simulink model "Noordergraaf_Rideout"  (R2022b)
settings: Solver=FixedStepAuto  StartTime=0.0  StopTime=stop_time  FixedStep=sample_time  RelTol=1e-3
InitFcn:
  | init_fcn_noordergraaf_rideout
StopFcn:
  | stop_fcn_noordergraaf_rideout
undefined symbols (not defined in the file): C, Cep, Cev, Cla, Cpa, Cpp, Cpv, Cra, Csa, Csp, Csv, Dx, fcs0, fes0, fes1, fesmin, fev0, fev1, fmax, fmin, Gx, initx, ka, KElv, KErv, kes, kev, KRlv, KRrv, ksys, L, Lpa, Lsa, P0lv, P0rv, Pn, R, R_105, R_26, R_29, R_34, R_35, R_60, R_61, R_64, R_65, R_66, R_70, R_82, R_84, R_88, R_90, R_AT, R_SA, Rev, Rla, Rpa, Rpp, Rpv, Rra ... (+18)
libraries: ee_lib x419, fl_lib x77, nesl_utility x52, simulink x2
(part 9 of 9)

== system Noordergraaf_Rideout/RLC_97 ==
  Capacitor : ee_lib/Passive/Capacitor  cap_option=0  c=C F  Cvec=[1e-05, 1e-06] F  Vvec=[0, 10] V  CV_table_symmetry=1  f_vec=[1, 10] kHz  DFext_vec=[.8, 1.2]  enable_C_tol=0  C_tol=5  tol_distribution=1  nSigma=4  r=1e-6 Ohm  g=0 1/Ohm  averaging_period=0 s  enable_operating_limits=0  operating_limit_action=2  max_working_voltage_range=[-25, 25] V  power_rating=1 W  enable_faults=0  fault_action=1  Cscale_faulted=100  R_faulted=1e-3 Ohm  G_faulted=0 1/Ohm  tau_fault=1e-3 s  enable_temporal_fault=0  t_fault=1 s  enable_behavioral_fault=0  max_permissible_voltage_range=[-100, 100] V  t_fail_on_voltage=1 s  i_specify=off  i_priority=None  i=0 A  i_nominal_specify=off  i_nominal_unit=A  i_nominal_value=1  v_specify=off  v_priority=None  v=0 V  v_nominal_specify=off  v_nominal_unit=V  v_nominal_value=1  vc_specify=off  vc_priority=High  vc=0 V  vc_nominal_specify=off  vc_nominal_unit=V  vc_nominal_value=1
  Inductor : ee_lib/Passive/Inductor  l=L H  enable_L_tol=0  L_tol=20  tol_distribution=1  nSigma=4  r=0 Ohm  g=1e-9 1/Ohm  enable_operating_limits=0  operating_limit_action=2  max_working_current=1 A  power_rating=1 W  enable_faults=0  fault_action=1  lambdaPercent=50  k_faulted=0.9999  turnsShort=0  openCct=0  groundShort=0  groundShortG=0 1/Ohm  tau_fault=1e-3 s  enable_temporal_fault=0  t_fault=1 s  enable_behavioral_fault=0  max_permissible_voltage=100 V  n_fail_on_voltage=1  max_permissible_current=1 A  t_fail_on_current=1 s  i_L_specify=off  i_L_priority=High  i_L=0 A  i_L_nominal_specify=off  i_L_nominal_unit=A  i_L_nominal_value=1
  Resistor1 : ee_lib/Passive/Resistor  R=R Ohm  enable_R_tol=0  R_tol=5  tol_distribution=1  nSigma=4  enable_operating_limits=0  operating_limit_action=2  max_working_voltage=100 V  power_rating=1 W  enable_faults=0  fault_action=1  R_faulted=inf Ohm  enable_temporal_fault=0  t_fault=1 s  enable_behavioral_fault=0  max_permissible_current=1 A  t_fail_on_current=1 s  noise_mode=0  sample_time=1e-3 s  repeatability=1  auto_seed=1874010528  user_seed=0  Tdevice=25 degC  power_derating_T1=70 degC  power_derating_T2=155 degC  operating_temperature_range_vec=[-50, 150] degC  alpha=3.93e-3 1/K  Tmeas=25 degC  thermal_mass=100 J/K  temperature_specify=off  temperature_priority=High  temperature=298.15 K  temperature_nominal_specify=off  temperature_nominal_unit=K  temperature_nominal_value=1
  Out_A : PMIOPort  Side=Left
  Out_B : PMIOPort  Port=2  Side=Left
  In_A : PMIOPort  Port=3  Side=Right
  In_B : PMIOPort  Port=4  Side=Right
  connections:
  Capacitor/LConn1 -- Out_A/RConn1 -- Inductor/RConn1
  Resistor1/RConn1 -- Inductor/LConn1
  Out_B/RConn1 -- In_B/RConn1 -- Capacitor/RConn1
  Resistor1/LConn1 -- In_A/RConn1

== system Noordergraaf_Rideout/RLC_98 ==
  Capacitor : ee_lib/Passive/Capacitor  cap_option=0  c=C F  Cvec=[1e-05, 1e-06] F  Vvec=[0, 10] V  CV_table_symmetry=1  f_vec=[1, 10] kHz  DFext_vec=[.8, 1.2]  enable_C_tol=0  C_tol=5  tol_distribution=1  nSigma=4  r=1e-6 Ohm  g=0 1/Ohm  averaging_period=0 s  enable_operating_limits=0  operating_limit_action=2  max_working_voltage_range=[-25, 25] V  power_rating=1 W  enable_faults=0  fault_action=1  Cscale_faulted=100  R_faulted=1e-3 Ohm  G_faulted=0 1/Ohm  tau_fault=1e-3 s  enable_temporal_fault=0  t_fault=1 s  enable_behavioral_fault=0  max_permissible_voltage_range=[-100, 100] V  t_fail_on_voltage=1 s  i_specify=off  i_priority=None  i=0 A  i_nominal_specify=off  i_nominal_unit=A  i_nominal_value=1  v_specify=off  v_priority=None  v=0 V  v_nominal_specify=off  v_nominal_unit=V  v_nominal_value=1  vc_specify=off  vc_priority=High  vc=0 V  vc_nominal_specify=off  vc_nominal_unit=V  vc_nominal_value=1
  Inductor : ee_lib/Passive/Inductor  l=L H  enable_L_tol=0  L_tol=20  tol_distribution=1  nSigma=4  r=0 Ohm  g=1e-9 1/Ohm  enable_operating_limits=0  operating_limit_action=2  max_working_current=1 A  power_rating=1 W  enable_faults=0  fault_action=1  lambdaPercent=50  k_faulted=0.9999  turnsShort=0  openCct=0  groundShort=0  groundShortG=0 1/Ohm  tau_fault=1e-3 s  enable_temporal_fault=0  t_fault=1 s  enable_behavioral_fault=0  max_permissible_voltage=100 V  n_fail_on_voltage=1  max_permissible_current=1 A  t_fail_on_current=1 s  i_L_specify=off  i_L_priority=High  i_L=0 A  i_L_nominal_specify=off  i_L_nominal_unit=A  i_L_nominal_value=1
  Resistor1 : ee_lib/Passive/Resistor  R=R Ohm  enable_R_tol=0  R_tol=5  tol_distribution=1  nSigma=4  enable_operating_limits=0  operating_limit_action=2  max_working_voltage=100 V  power_rating=1 W  enable_faults=0  fault_action=1  R_faulted=inf Ohm  enable_temporal_fault=0  t_fault=1 s  enable_behavioral_fault=0  max_permissible_current=1 A  t_fail_on_current=1 s  noise_mode=0  sample_time=1e-3 s  repeatability=1  auto_seed=746693110  user_seed=0  Tdevice=25 degC  power_derating_T1=70 degC  power_derating_T2=155 degC  operating_temperature_range_vec=[-50, 150] degC  alpha=3.93e-3 1/K  Tmeas=25 degC  thermal_mass=100 J/K  temperature_specify=off  temperature_priority=High  temperature=298.15 K  temperature_nominal_specify=off  temperature_nominal_unit=K  temperature_nominal_value=1
  Out_A : PMIOPort  Side=Left
  Out_B : PMIOPort  Port=2  Side=Left
  In_A : PMIOPort  Port=3  Side=Right
  In_B : PMIOPort  Port=4  Side=Right
  connections:
  Capacitor/LConn1 -- Out_A/RConn1 -- Inductor/RConn1
  Resistor1/RConn1 -- Inductor/LConn1
  Out_B/RConn1 -- In_B/RConn1 -- Capacitor/RConn1
  Resistor1/LConn1 -- In_A/RConn1

== system Noordergraaf_Rideout/RLC_99 ==
  Capacitor : ee_lib/Passive/Capacitor  cap_option=0  c=C F  Cvec=[1e-05, 1e-06] F  Vvec=[0, 10] V  CV_table_symmetry=1  f_vec=[1, 10] kHz  DFext_vec=[.8, 1.2]  enable_C_tol=0  C_tol=5  tol_distribution=1  nSigma=4  r=1e-6 Ohm  g=0 1/Ohm  averaging_period=0 s  enable_operating_limits=0  operating_limit_action=2  max_working_voltage_range=[-25, 25] V  power_rating=1 W  enable_faults=0  fault_action=1  Cscale_faulted=100  R_faulted=1e-3 Ohm  G_faulted=0 1/Ohm  tau_fault=1e-3 s  enable_temporal_fault=0  t_fault=1 s  enable_behavioral_fault=0  max_permissible_voltage_range=[-100, 100] V  t_fail_on_voltage=1 s  i_specify=off  i_priority=None  i=0 A  i_nominal_specify=off  i_nominal_unit=A  i_nominal_value=1  v_specify=off  v_priority=None  v=0 V  v_nominal_specify=off  v_nominal_unit=V  v_nominal_value=1  vc_specify=off  vc_priority=High  vc=0 V  vc_nominal_specify=off  vc_nominal_unit=V  vc_nominal_value=1
  Inductor : ee_lib/Passive/Inductor  l=L H  enable_L_tol=0  L_tol=20  tol_distribution=1  nSigma=4  r=0 Ohm  g=1e-9 1/Ohm  enable_operating_limits=0  operating_limit_action=2  max_working_current=1 A  power_rating=1 W  enable_faults=0  fault_action=1  lambdaPercent=50  k_faulted=0.9999  turnsShort=0  openCct=0  groundShort=0  groundShortG=0 1/Ohm  tau_fault=1e-3 s  enable_temporal_fault=0  t_fault=1 s  enable_behavioral_fault=0  max_permissible_voltage=100 V  n_fail_on_voltage=1  max_permissible_current=1 A  t_fail_on_current=1 s  i_L_specify=off  i_L_priority=High  i_L=0 A  i_L_nominal_specify=off  i_L_nominal_unit=A  i_L_nominal_value=1
  Resistor1 : ee_lib/Passive/Resistor  R=R Ohm  enable_R_tol=0  R_tol=5  tol_distribution=1  nSigma=4  enable_operating_limits=0  operating_limit_action=2  max_working_voltage=100 V  power_rating=1 W  enable_faults=0  fault_action=1  R_faulted=inf Ohm  enable_temporal_fault=0  t_fault=1 s  enable_behavioral_fault=0  max_permissible_current=1 A  t_fail_on_current=1 s  noise_mode=0  sample_time=1e-3 s  repeatability=1  auto_seed=112129176  user_seed=0  Tdevice=25 degC  power_derating_T1=70 degC  power_derating_T2=155 degC  operating_temperature_range_vec=[-50, 150] degC  alpha=3.93e-3 1/K  Tmeas=25 degC  thermal_mass=100 J/K  temperature_specify=off  temperature_priority=High  temperature=298.15 K  temperature_nominal_specify=off  temperature_nominal_unit=K  temperature_nominal_value=1
  Out_A : PMIOPort  Side=Left
  Out_B : PMIOPort  Port=2  Side=Left
  In_A : PMIOPort  Port=3  Side=Right
  In_B : PMIOPort  Port=4  Side=Right
  connections:
  Capacitor/LConn1 -- Out_A/RConn1 -- Inductor/RConn1
  Resistor1/RConn1 -- Inductor/LConn1
  Out_B/RConn1 -- In_B/RConn1 -- Capacitor/RConn1
  Resistor1/LConn1 -- In_A/RConn1

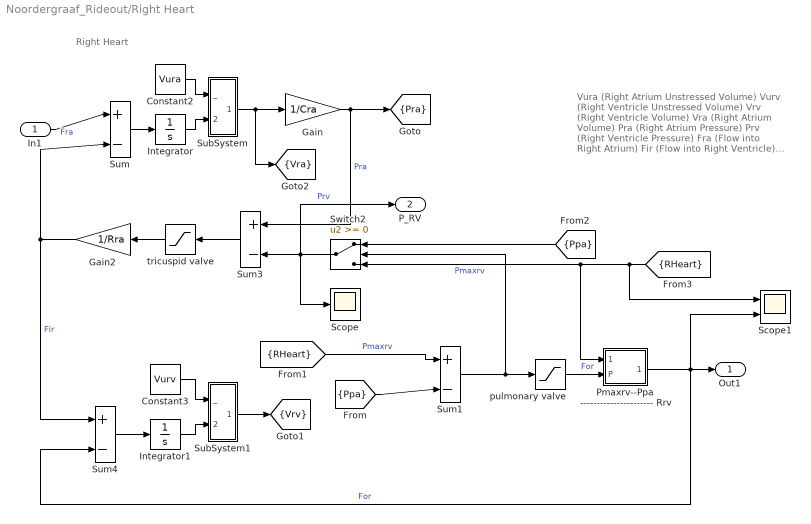
== system Noordergraaf_Rideout/Right Heart ==
  note: Right Heart
  note: Vura (Right Atrium Unstressed Volume)
      | Vurv (Right Ventricle Unstressed Volume)
      | Vrv (Right Ventricle Volume)
      | Vra (Right Atrium Volume)
      | Pra (Right Atrium Pressure)
      | Prv (Right Ventricle Pressure)
      | Fra (Flow into Right Atrium)
      | Fir (Flow into Right Ventricle)
      | For (Flow out of Right Ventricle)
      | LHeart (Left Ventricle Function)
  In1 : Inport
  Constant2 : Constant  Value=Vura
  Constant3 : Constant  Value=Vurv
  Gain : Gain  Gain=1/Cra  SaturateOnIntegerOverflow=on
  Gain2 : Gain  Gain=1/Rra  SaturateOnIntegerOverflow=on
  Integrator : Integrator
  Integrator1 : Integrator
  Pmaxrv--Ppa ---------------------- Rrv : Subsystem
  Scope : Scope
  Scope1 : Scope  NumInputPorts=2
  SubSystem : Subsystem
  SubSystem1 : Subsystem
  Sum : Sum  Inputs=|+-  SaturateOnIntegerOverflow=on
  Sum1 : Sum  Inputs=|+-  SaturateOnIntegerOverflow=on
  Sum3 : Sum  Inputs=+-  SaturateOnIntegerOverflow=on
  Sum4 : Sum  Inputs=+-  SaturateOnIntegerOverflow=on
  Switch2 : Switch
  pulmonary valve : Saturate  UpperLimit=inf  LowerLimit=0
  tricuspid valve : Saturate  UpperLimit=inf  LowerLimit=0
  Out1 : Outport
  P_RV : Outport  Port=2
  tag scope: Pra=scoped, Vra=scoped, Vrv=scoped
  wires:
  In1/1 -> Sum/1  "Fra"
  Sum/1 -> Integrator/1
  [Ppa] -> Sum1/2
  Gain/1 -> [Pra], Sum3/1  "Pra"
  Gain2/1 -> Sum/2, Sum4/1  "Fir"
  Integrator/1 -> SubSystem/2(+)
  Constant2/1 -> SubSystem/1(_)
  SubSystem1/1(Out) -> [Vrv]
  SubSystem/1(Out) -> Gain/1, [Vra]
  Constant3/1 -> SubSystem1/1(_)
  Integrator1/1 -> SubSystem1/2(+)
  [RHeart] -> Sum1/1  "Pmaxrv"
  Sum1/1 -> pulmonary valve/1, Switch2/2
  [Ppa] -> Switch2/1
  tricuspid valve/1 -> Gain2/1
  pulmonary valve/1 -> Pmaxrv--Ppa ---------------------- Rrv/2(P)  "For"
  Pmaxrv--Ppa ---------------------- Rrv/1(Flow) -> Scope1/2, Out1/1, Sum4/2  "For"
  [RHeart] -> Scope1/1, Switch2/3, Pmaxrv--Ppa ---------------------- Rrv/1(Pmax)  "Pmaxrv"
  Sum4/1 -> Integrator1/1
  Sum3/1 -> tricuspid valve/1
  Switch2/1 -> P_RV/1, Sum3/2, Scope/1  "Prv"

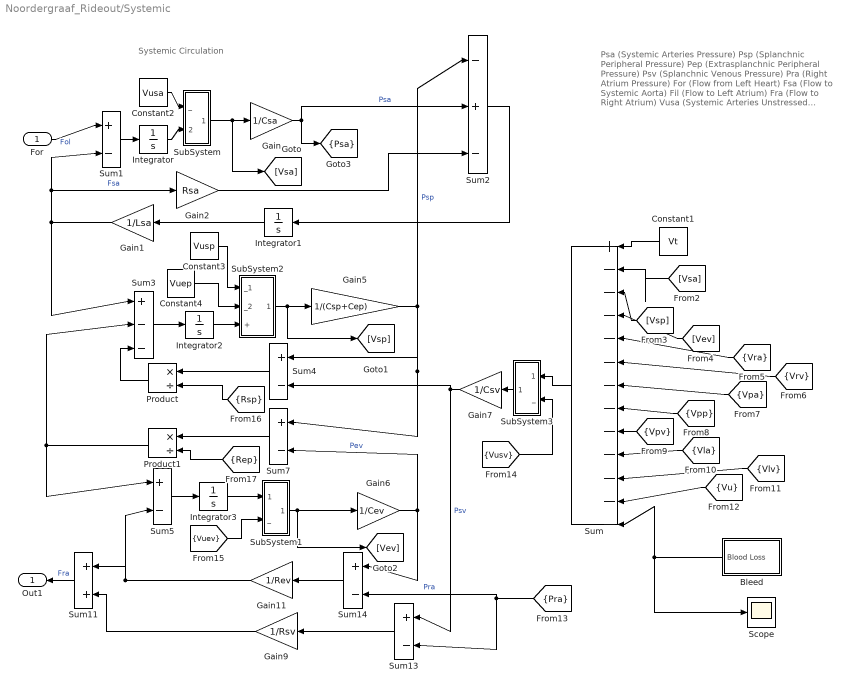
== system Noordergraaf_Rideout/Systemic ==
  note: Psa (Systemic Arteries Pressure)
      | Psp (Splanchnic Peripheral Pressure)
      | Pep (Extrasplanchnic Peripheral Pressure)
      | Psv (Splanchnic Venous Pressure)
      | Pra (Right Atrium Pressure)
      | For (Flow from Left Heart)
      | Fsa (Flow to Systemic Aorta)
      | Fil (Flow to Left Atrium)
      | Fra (Flow to Right Atrium)
      | Vusa (Systemic Arteries Unstressed Volume)
      | Vusp (Extrasplanchnic Venous Unstressed Volume)
      | Vuep (Splanchnic Venous Unstressed Volume)
      | Vuev (Extrasplanchnic Venous Unstressed Volume)
      | Vusv (Splanchnic Venous Unstressed Volume)
  note: Systemic Circulation
  For : Inport
  Bleed : Subsystem  mask{ulimit=0, rate=0, tstart=0}
      mask prompts: ulimit "Bleed Up Limit (ml)"; rate "Bleed Rate (ml/s)"; tstart "Bleed Start Time (s)"
  Constant1 : Constant  Value=Vt
  Constant2 : Constant  Value=Vusa
  Constant3 : Constant  Value=Vusp
  Constant4 : Constant  Value=Vuep
  Gain : Gain  Gain=1/Csa  SaturateOnIntegerOverflow=on
  Gain1 : Gain  Gain=1/Lsa  SaturateOnIntegerOverflow=on
  Gain11 : Gain  Gain=1/Rev  SaturateOnIntegerOverflow=on
  Gain2 : Gain  Gain=Rsa  SaturateOnIntegerOverflow=on
  Gain5 : Gain  Gain=1/(Csp+Cep)  SaturateOnIntegerOverflow=on
  Gain6 : Gain  Gain=1/Cev  SaturateOnIntegerOverflow=on
  Gain7 : Gain  Gain=1/Csv  SaturateOnIntegerOverflow=on
  Gain9 : Gain  Gain=1/Rsv  SaturateOnIntegerOverflow=on
  Integrator{,1..3} (4 alike) : Integrator
  Product : Product  Inputs=*/  SaturateOnIntegerOverflow=on
  Product1 : Product  Inputs=*/  SaturateOnIntegerOverflow=on
  Scope : Scope
  SubSystem : Subsystem
  SubSystem1 : Subsystem
  SubSystem2 : Subsystem
  SubSystem3 : Subsystem
  Sum : Sum  Inputs=|+------------  SaturateOnIntegerOverflow=on
  Sum{1,4..5,7,13..14} (6 alike) : Sum  Inputs=|+-  SaturateOnIntegerOverflow=on
  Sum11 : Sum  Inputs=|++  SaturateOnIntegerOverflow=on
  Sum2 : Sum  Inputs=|-+-  SaturateOnIntegerOverflow=on
  Sum3 : Sum  Inputs=|+--  SaturateOnIntegerOverflow=on
  Out1 : Outport
  tag scope: Psa=scoped
  wires:
  For/1 -> Sum1/1  "Fol"
  Sum1/1 -> Integrator/1
  Integrator1/1 -> Gain1/1
  Sum2/1 -> Integrator1/1
  Gain2/1 -> Sum2/3
  Gain1/1 -> Sum1/2, Gain2/1, Sum3/1  "Fsa"
  Sum3/1 -> Integrator2/1
  Gain5/1 -> Sum2/1, Sum4/1, Sum7/1  "Psp"
  Product/1 -> Sum3/3
  Product1/1 -> Sum3/2, Sum5/1
  Integrator3/1 -> SubSystem1/1(+)
  SubSystem1/1(Out) -> Gain6/1, [Vev]
  Constant1/1 -> Sum/1
  [Vsa] -> Sum/2
  [Vsp] -> Sum/3
  [Vev] -> Sum/4
  [Vra] -> Sum/5
  [Vrv] -> Sum/6
  [Vpa] -> Sum/7
  [Vpp] -> Sum/8
  [Vpv] -> Sum/9
  [Vla] -> Sum/10
  [Vlv] -> Sum/11
  [Vu] -> Sum/12
  Integrator/1 -> SubSystem/2(+)
  SubSystem/1(Out) -> Gain/1, [Vsa]
  Integrator2/1 -> SubSystem2/3(+)
  SubSystem2/1(Out) -> Gain5/1, [Vsp]
  SubSystem3/1(Out) -> Gain7/1
  Sum13/1 -> Gain9/1
  Sum11/1 -> Out1/1  "Fra"
  Gain7/1 -> Sum4/2, Sum13/1  "Psv"
  Gain9/1 -> Sum11/2
  Gain6/1 -> Sum7/2, Sum14/1  "Pev"
  Sum14/1 -> Gain11/1
  [Pra] -> Sum13/2, Sum14/2  "Pra"
  Sum5/1 -> Integrator3/1
  Gain11/1 -> Sum11/1, Sum5/2
  Gain/1 -> [Psa], Sum2/2  "Psa"
  Constant2/1 -> SubSystem/1(_)
  [Vuev] -> SubSystem1/2(_)
  Constant3/1 -> SubSystem2/1(_1)
  Constant4/1 -> SubSystem2/2(_2)
  Sum/1 -> SubSystem3/1(+)
  [Vusv] -> SubSystem3/2(_)
  Sum4/1 -> Product/1
  [Rsp] -> Product/2
  [Rep] -> Product1/2
  Sum7/1 -> Product1/1
  Bleed/1(Blood Loss) -> Sum/13, Scope/1

== system Noordergraaf_Rideout/Voltage Source (SL) ==
  S : Inport
  Controlled Voltage Source : fl_lib/Electrical/Electrical Sources/Controlled Voltage Source
  Simulink-PS Converter : nesl_utility/Simulink-PS Converter  PhysicalDomain=network_engine_domain  SubClassName=ps_input  LeftPortType=input  RightPortType=output  PseudoPeriodic=off  Frequencies=[]  NoiseDistribution=none  NoiseParameters=[]  Unit=V  AffineConversion=off  FilteringAndDerivatives=zero  SimscapeFilterOrder=1  InputFilterTimeConstant=.001  UdotUserProvided=0
  + : PMIOPort  Side=Right
  - : PMIOPort  Port=2  Side=Right
  wires:
  S/1 -> Simulink-PS Converter/1
  connections:
  +/RConn1 -- Controlled Voltage Source/LConn1
  -/RConn1 -- Controlled Voltage Source/RConn2
  Controlled Voltage Source/RConn1 -- Simulink-PS Converter/RConn1

== system Noordergraaf_Rideout/Control/Carotid Sinus ==
  Pin : Inport
  Fcn : Fcn  Expr=(fmin+fmax*exp((u-Pn)/ka))/(1+exp((u-Pn)/ka))
  Transfer Fcn : TransferFcn  Numerator=[touz 1]  Denominator=[toup 1]
  fcs : Outport
  wires:
  Pin/1 -> Transfer Fcn/1
  Transfer Fcn/1 -> Fcn/1
  Fcn/1 -> fcs/1

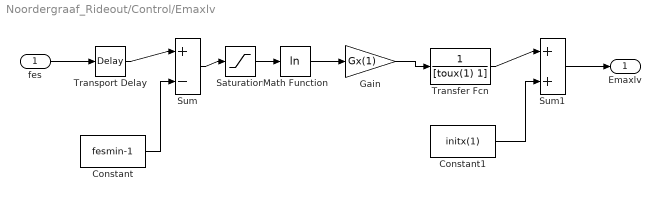
== system Noordergraaf_Rideout/Control/Emaxlv ==
  fes : Inport
  Constant : Constant  Value=fesmin-1
  Constant1 : Constant  Value=initx(1)
  Gain : Gain  Gain=Gx(1)  SaturateOnIntegerOverflow=on
  Math Function : Math  Operator=log
  Saturation : Saturate  UpperLimit=inf  LowerLimit=1
  Sum : Sum  Inputs=|+-  SaturateOnIntegerOverflow=on
  Sum1 : Sum  Inputs=|++  SaturateOnIntegerOverflow=on
  Transfer Fcn : TransferFcn  Denominator=[toux(1) 1]
  Transport Delay : TransportDelay  DelayTime=Dx(1)
  Emaxlv : Outport
  wires:
  fes/1 -> Transport Delay/1
  Transport Delay/1 -> Sum/1
  Constant/1 -> Sum/2
  Sum/1 -> Saturation/1
  Saturation/1 -> Math Function/1
  Math Function/1 -> Gain/1
  Gain/1 -> Transfer Fcn/1
  Transfer Fcn/1 -> Sum1/1
  Sum1/1 -> Emaxlv/1
  Constant1/1 -> Sum1/2

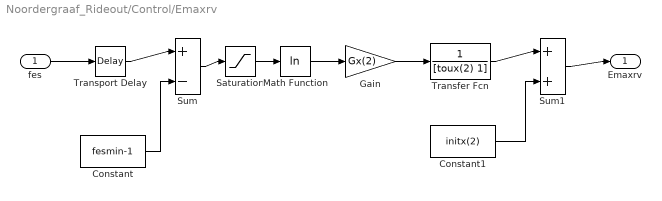
== system Noordergraaf_Rideout/Control/Emaxrv ==
  fes : Inport
  Constant : Constant  Value=fesmin-1
  Constant1 : Constant  Value=initx(2)
  Gain : Gain  Gain=Gx(2)  SaturateOnIntegerOverflow=on
  Math Function : Math  Operator=log
  Saturation : Saturate  UpperLimit=inf  LowerLimit=1
  Sum : Sum  Inputs=|+-  SaturateOnIntegerOverflow=on
  Sum1 : Sum  Inputs=|++  SaturateOnIntegerOverflow=on
  Transfer Fcn : TransferFcn  Denominator=[toux(2) 1]
  Transport Delay : TransportDelay  DelayTime=Dx(2)
  Emaxrv : Outport
  wires:
  Constant1/1 -> Sum1/2
  Sum1/1 -> Emaxrv/1
  Transfer Fcn/1 -> Sum1/1
  Gain/1 -> Transfer Fcn/1
  Math Function/1 -> Gain/1
  Saturation/1 -> Math Function/1
  Sum/1 -> Saturation/1
  Constant/1 -> Sum/2
  Transport Delay/1 -> Sum/1
  fes/1 -> Transport Delay/1

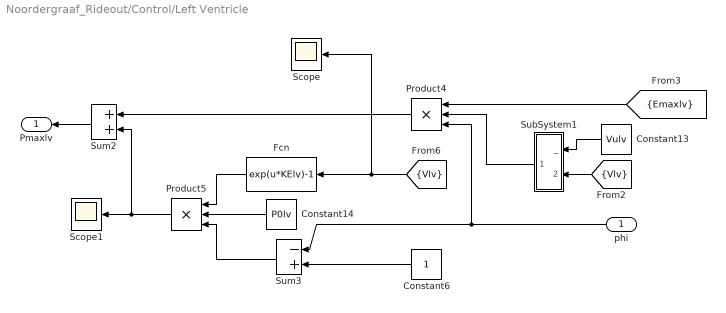
== system Noordergraaf_Rideout/Control/Left Ventricle ==
  phi : Inport
  Constant13 : Constant  Value=Vulv
  Constant14 : Constant  Value=P0lv
  Constant6 : Constant
  Fcn : Fcn  Expr=exp(u*KElv)-1
  Product4 : Product  Inputs=3  SaturateOnIntegerOverflow=on
  Product5 : Product  Inputs=3  SaturateOnIntegerOverflow=on
  Scope : Scope
  Scope1 : Scope
  SubSystem1 : Subsystem
  Sum2 : Sum  SaturateOnIntegerOverflow=on
  Sum3 : Sum  Inputs=-+  SaturateOnIntegerOverflow=on
  Pmaxlv : Outport
  wires:
  Sum2/1 -> Pmaxlv/1
  Product4/1 -> Sum2/1
  Product5/1 -> Sum2/2, Scope1/1
  Fcn/1 -> Product5/1
  Constant14/1 -> Product5/2
  Sum3/1 -> Product5/3
  Constant6/1 -> Sum3/2
  Constant13/1 -> SubSystem1/1(_)
  [Vlv] -> SubSystem1/2(+)
  SubSystem1/1(Out) -> Product4/2
  phi/1 -> Sum3/1, Product4/3
  [Emaxlv] -> Product4/1
  [Vlv] -> Fcn/1, Scope/1

== system Noordergraaf_Rideout/Control/Rep ==
  fes : Inport
  Constant : Constant  Value=fesmin-1
  Constant1 : Constant  Value=initx(4)
  Gain : Gain  Gain=Gx(4)  SaturateOnIntegerOverflow=on
  Math Function : Math  Operator=log
  Saturation : Saturate  UpperLimit=inf  LowerLimit=1
  Sum : Sum  Inputs=|+-  SaturateOnIntegerOverflow=on
  Sum1 : Sum  Inputs=|++  SaturateOnIntegerOverflow=on
  Transfer Fcn : TransferFcn  Denominator=[toux(4) 1]
  Transport Delay : TransportDelay  DelayTime=Dx(4)
  Rep : Outport
  wires:
  Constant1/1 -> Sum1/2
  Sum1/1 -> Rep/1
  Transfer Fcn/1 -> Sum1/1
  Gain/1 -> Transfer Fcn/1
  Math Function/1 -> Gain/1
  Saturation/1 -> Math Function/1
  Sum/1 -> Saturation/1
  Constant/1 -> Sum/2
  Transport Delay/1 -> Sum/1
  fes/1 -> Transport Delay/1

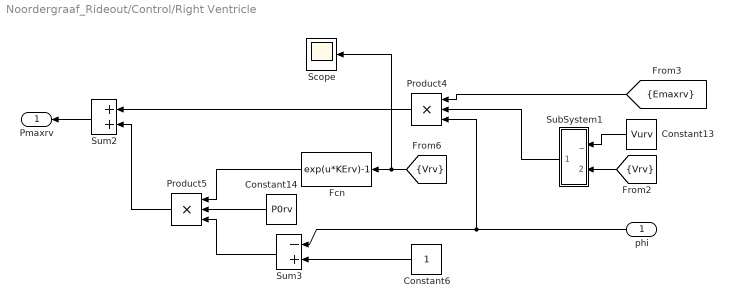
== system Noordergraaf_Rideout/Control/Right Ventricle ==
  phi : Inport
  Constant13 : Constant  Value=Vurv
  Constant14 : Constant  Value=P0rv
  Constant6 : Constant
  Fcn : Fcn  Expr=exp(u*KErv)-1
  Product4 : Product  Inputs=3  SaturateOnIntegerOverflow=on
  Product5 : Product  Inputs=3  SaturateOnIntegerOverflow=on
  Scope : Scope
  SubSystem1 : Subsystem
  Sum2 : Sum  SaturateOnIntegerOverflow=on
  Sum3 : Sum  Inputs=-+  SaturateOnIntegerOverflow=on
  Pmaxrv : Outport
  wires:
  Constant6/1 -> Sum3/2
  Sum3/1 -> Product5/3
  Constant14/1 -> Product5/2
  Fcn/1 -> Product5/1
  Product5/1 -> Sum2/2
  Product4/1 -> Sum2/1
  Sum2/1 -> Pmaxrv/1
  [Emaxrv] -> Product4/1
  [Vrv] -> SubSystem1/2(+)
  Constant13/1 -> SubSystem1/1(_)
  SubSystem1/1(Out) -> Product4/2
  phi/1 -> Sum3/1, Product4/3
  [Vrv] -> Fcn/1, Scope/1

== system Noordergraaf_Rideout/Control/Rsp ==
  fes : Inport
  Constant : Constant  Value=fesmin-1
  Constant1 : Constant  Value=initx(3)
  Gain : Gain  Gain=Gx(3)  SaturateOnIntegerOverflow=on
  Math Function : Math  Operator=log
  Saturation : Saturate  UpperLimit=inf  LowerLimit=1
  Sum : Sum  Inputs=|+-  SaturateOnIntegerOverflow=on
  Sum1 : Sum  Inputs=|++  SaturateOnIntegerOverflow=on
  Transfer Fcn : TransferFcn  Denominator=[toux(3) 1]
  Transport Delay : TransportDelay  DelayTime=Dx(3)
  Rsp : Outport
  wires:
  fes/1 -> Transport Delay/1
  Transport Delay/1 -> Sum/1
  Constant/1 -> Sum/2
  Sum/1 -> Saturation/1
  Saturation/1 -> Math Function/1
  Math Function/1 -> Gain/1
  Gain/1 -> Transfer Fcn/1
  Transfer Fcn/1 -> Sum1/1
  Sum1/1 -> Rsp/1
  Constant1/1 -> Sum1/2

== system Noordergraaf_Rideout/Control/Sympathetic Pathway ==
  fcs : Inport
  Constant : Constant  Value=fes1
  Gain : Gain  Gain=-kes  SaturateOnIntegerOverflow=on
  Gain1 : Gain  Gain=fes0-fes1  SaturateOnIntegerOverflow=on
  Math Function : Math
  Sum : Sum  Inputs=|++  SaturateOnIntegerOverflow=on
  fes : Outport
  wires:
  Gain1/1 -> Sum/1
  Constant/1 -> Sum/2
  Sum/1 -> fes/1
  fcs/1 -> Gain/1
  Gain/1 -> Math Function/1
  Math Function/1 -> Gain1/1

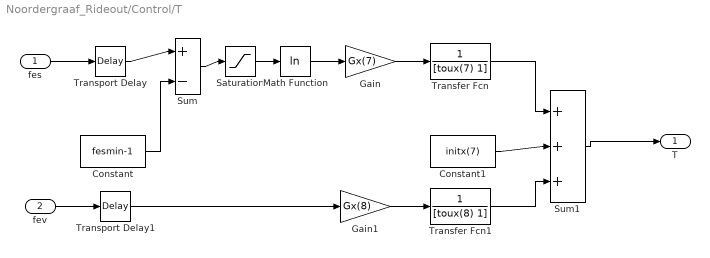
== system Noordergraaf_Rideout/Control/T ==
  fes : Inport
  fev : Inport  Port=2
  Constant : Constant  Value=fesmin-1
  Constant1 : Constant  Value=initx(7)
  Gain : Gain  Gain=Gx(7)  SaturateOnIntegerOverflow=on
  Gain1 : Gain  Gain=Gx(8)  SaturateOnIntegerOverflow=on
  Math Function : Math  Operator=log
  Saturation : Saturate  UpperLimit=inf  LowerLimit=1
  Sum : Sum  Inputs=|+-  SaturateOnIntegerOverflow=on
  Sum1 : Sum  Inputs=|+++  SaturateOnIntegerOverflow=on
  Transfer Fcn : TransferFcn  Denominator=[toux(7) 1]
  Transfer Fcn1 : TransferFcn  Denominator=[toux(8) 1]
  Transport Delay : TransportDelay  DelayTime=Dx(7)
  Transport Delay1 : TransportDelay  DelayTime=Dx(8)
  T : Outport
  wires:
  fes/1 -> Transport Delay/1
  Transport Delay/1 -> Sum/1
  Constant/1 -> Sum/2
  Sum/1 -> Saturation/1
  Saturation/1 -> Math Function/1
  Math Function/1 -> Gain/1
  Gain/1 -> Transfer Fcn/1
  Transfer Fcn/1 -> Sum1/1
  Sum1/1 -> T/1
  Constant1/1 -> Sum1/2
  fev/1 -> Transport Delay1/1
  Transport Delay1/1 -> Gain1/1
  Gain1/1 -> Transfer Fcn1/1
  Transfer Fcn1/1 -> Sum1/3

== system Noordergraaf_Rideout/Control/Vagal Pathway ==
  fcs : Inport
  Fcn : Fcn  Expr=(fev0+fev1*exp((u-fcs0)/kev))/(1+exp((u-fcs0)/kev))
  fev : Outport
  wires:
  Fcn/1 -> fev/1
  fcs/1 -> Fcn/1

== system Noordergraaf_Rideout/Control/Vuev ==
  fes : Inport
  Constant : Constant  Value=fesmin-1
  Constant1 : Constant  Value=initx(6)
  Gain : Gain  Gain=Gx(6)  SaturateOnIntegerOverflow=on
  Math Function : Math  Operator=log
  Saturation : Saturate  UpperLimit=inf  LowerLimit=1
  Sum : Sum  Inputs=|+-  SaturateOnIntegerOverflow=on
  Sum1 : Sum  Inputs=|++  SaturateOnIntegerOverflow=on
  Transfer Fcn : TransferFcn  Denominator=[toux(6) 1]
  Transport Delay : TransportDelay  DelayTime=Dx(6)
  Vuev : Outport
  wires:
  Constant1/1 -> Sum1/2
  Sum1/1 -> Vuev/1
  Transfer Fcn/1 -> Sum1/1
  Gain/1 -> Transfer Fcn/1
  Math Function/1 -> Gain/1
  Saturation/1 -> Math Function/1
  Sum/1 -> Saturation/1
  Constant/1 -> Sum/2
  Transport Delay/1 -> Sum/1
  fes/1 -> Transport Delay/1

== system Noordergraaf_Rideout/Control/Vusv ==
  fes : Inport
  Constant : Constant  Value=fesmin-1
  Constant1 : Constant  Value=initx(5)
  Gain : Gain  Gain=Gx(5)  SaturateOnIntegerOverflow=on
  Math Function : Math  Operator=log
  Saturation : Saturate  UpperLimit=inf  LowerLimit=1
  Sum : Sum  Inputs=|+-  SaturateOnIntegerOverflow=on
  Sum1 : Sum  Inputs=|++  SaturateOnIntegerOverflow=on
  Transfer Fcn : TransferFcn  Denominator=[toux(5) 1]
  Transport Delay : TransportDelay  DelayTime=Dx(5)
  Vusv : Outport
  wires:
  fes/1 -> Transport Delay/1
  Transport Delay/1 -> Sum/1
  Constant/1 -> Sum/2
  Sum/1 -> Saturation/1
  Saturation/1 -> Math Function/1
  Math Function/1 -> Gain/1
  Gain/1 -> Transfer Fcn/1
  Transfer Fcn/1 -> Sum1/1
  Sum1/1 -> Vusv/1
  Constant1/1 -> Sum1/2

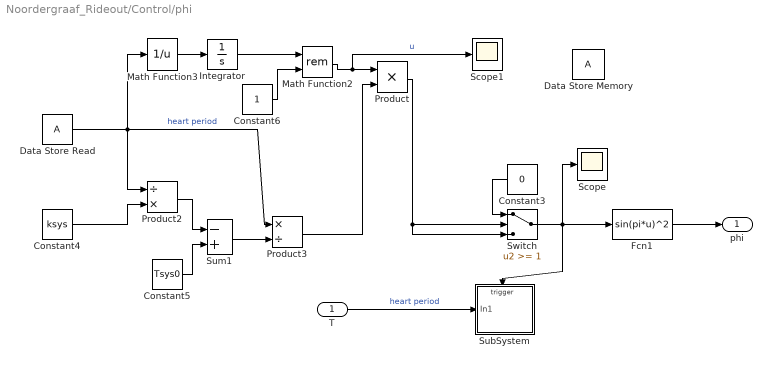
== system Noordergraaf_Rideout/Control/phi ==
  T : Inport
  Constant3 : Constant  Value=0
  Constant4 : Constant  Value=ksys
  Constant5 : Constant  Value=Tsys0
  Constant6 : Constant
  Data Store Memory : DataStoreMemory  InitialValue=initx(7)  ShowAdditionalParam=off
  Data Store Read : DataStoreRead  SampleTime=0  IndexOptions=Index vector (dialog)  Indices=1  OutputSizes=1
  Fcn1 : Fcn  Expr=sin(pi*u)^2
  Integrator : Integrator
  Math Function2 : Math  Operator=rem
  Math Function3 : Math  Operator=reciprocal
  Product : Product  SaturateOnIntegerOverflow=on
  Product2 : Product  Inputs=/*  SaturateOnIntegerOverflow=on
  Product3 : Product  Inputs=*/  SaturateOnIntegerOverflow=on
  Scope : Scope
  Scope1 : Scope
  SubSystem : Subsystem  TreatAsAtomicUnit=on
  Sum1 : Sum  Inputs=-+  SaturateOnIntegerOverflow=on
  Switch : Switch  Threshold=1
  phi : Outport
  wires:
  Product3/1 -> Product/2
  Sum1/1 -> Product3/2
  Constant5/1 -> Sum1/2
  Product2/1 -> Sum1/1
  Constant4/1 -> Product2/2
  Constant3/1 -> Switch/1
  Product/1 -> Switch/2, Switch/3
  Fcn1/1 -> phi/1
  T/1 -> SubSystem/1(In1)  "heart period"
  Switch/1 -> Fcn1/1, SubSystem/Trigger, Scope/1
  Data Store Read/1 -> Product3/1, Product2/1, Math Function3/1  "heart period"
  Constant6/1 -> Math Function2/2
  Math Function2/1 -> Product/1, Scope1/1  "u"
  Math Function3/1 -> Integrator/1
  Integrator/1 -> Math Function2/1

== system Noordergraaf_Rideout/Left Heart/Pmaxlv--Psa ---------------------- Rlv ==
  Pmax : Inport
  P : Inport  Port=2
  Gain : Gain  Gain=KRlv  SaturateOnIntegerOverflow=on
  Product : Product  Inputs=/*  SaturateOnIntegerOverflow=on
  Saturation : Saturate  UpperLimit=inf  LowerLimit=0.01
  Flow : Outport
  wires:
  Pmax/1 -> Gain/1
  Gain/1 -> Saturation/1
  P/1 -> Product/2
  Saturation/1 -> Product/1
  Product/1 -> Flow/1

== system Noordergraaf_Rideout/Left Heart/SubSystem ==
  _ : Inport
  + : Inport  Port=2
  Saturation : Saturate  UpperLimit=10000  LowerLimit=0
  Sum : Sum  Inputs=|-+  SaturateOnIntegerOverflow=on
  Out : Outport
  wires:
  _/1 -> Sum/1
  +/1 -> Sum/2
  Sum/1 -> Saturation/1
  Saturation/1 -> Out/1

== system Noordergraaf_Rideout/Left Heart/SubSystem1 ==
  _ : Inport
  + : Inport  Port=2
  Saturation : Saturate  UpperLimit=10000  LowerLimit=0
  Sum : Sum  Inputs=|-+  SaturateOnIntegerOverflow=on
  Out : Outport
  wires:
  Saturation/1 -> Out/1
  Sum/1 -> Saturation/1
  +/1 -> Sum/2
  _/1 -> Sum/1

== system Noordergraaf_Rideout/Pulmonary/SubSystem ==
  _ : Inport
  + : Inport  Port=2
  Saturation : Saturate  UpperLimit=10000  LowerLimit=0
  Sum : Sum  Inputs=|-+  SaturateOnIntegerOverflow=on
  Out : Outport
  wires:
  _/1 -> Sum/1
  +/1 -> Sum/2
  Sum/1 -> Saturation/1
  Saturation/1 -> Out/1

== system Noordergraaf_Rideout/Pulmonary/SubSystem1 ==
  _ : Inport
  + : Inport  Port=2
  Saturation : Saturate  UpperLimit=10000  LowerLimit=0
  Sum : Sum  Inputs=|-+  SaturateOnIntegerOverflow=on
  Out : Outport
  wires:
  _/1 -> Sum/1
  +/1 -> Sum/2
  Sum/1 -> Saturation/1
  Saturation/1 -> Out/1

== system Noordergraaf_Rideout/Pulmonary/SubSystem2 ==
  _ : Inport
  + : Inport  Port=2
  Saturation : Saturate  UpperLimit=10000  LowerLimit=0
  Sum : Sum  Inputs=|-+  SaturateOnIntegerOverflow=on
  Out : Outport
  wires:
  Saturation/1 -> Out/1
  Sum/1 -> Saturation/1
  +/1 -> Sum/2
  _/1 -> Sum/1

== system Noordergraaf_Rideout/Right Heart/Pmaxrv--Ppa ---------------------- Rrv ==
  Pmax : Inport
  P : Inport  Port=2
  Gain : Gain  Gain=KRrv  SaturateOnIntegerOverflow=on
  Product : Product  Inputs=/*  SaturateOnIntegerOverflow=on
  Saturation : Saturate  UpperLimit=inf  LowerLimit=0.01
  Flow : Outport
  wires:
  Pmax/1 -> Gain/1
  Gain/1 -> Saturation/1
  P/1 -> Product/2
  Saturation/1 -> Product/1
  Product/1 -> Flow/1

== system Noordergraaf_Rideout/Right Heart/SubSystem ==
  _ : Inport
  + : Inport  Port=2
  Saturation : Saturate  UpperLimit=10000  LowerLimit=0
  Sum : Sum  Inputs=|-+  SaturateOnIntegerOverflow=on
  Out : Outport
  wires:
  _/1 -> Sum/1
  +/1 -> Sum/2
  Sum/1 -> Saturation/1
  Saturation/1 -> Out/1

== system Noordergraaf_Rideout/Right Heart/SubSystem1 ==
  _ : Inport
  + : Inport  Port=2
  Saturation : Saturate  UpperLimit=10000  LowerLimit=0
  Sum : Sum  Inputs=|-+  SaturateOnIntegerOverflow=on
  Out : Outport
  wires:
  Saturation/1 -> Out/1
  Sum/1 -> Saturation/1
  +/1 -> Sum/2
  _/1 -> Sum/1

== system Noordergraaf_Rideout/Systemic/Bleed ==
  Clock : Clock
  Constant : Constant  Value=0
  Ramp : simulink/Sources/Ramp  slope=rate  start=tstart  InitialOutput=0
  Saturation : Saturate  UpperLimit=ulimit  LowerLimit=0
  Switch : Switch  Threshold=tstart
  Blood Loss : Outport
  wires:
  Clock/1 -> Switch/2
  Constant/1 -> Switch/3
  Ramp/1 -> Switch/1
  Switch/1 -> Saturation/1
  Saturation/1 -> Blood Loss/1

== system Noordergraaf_Rideout/Systemic/SubSystem ==
  _ : Inport
  + : Inport  Port=2
  Saturation : Saturate  UpperLimit=10000  LowerLimit=0
  Sum : Sum  Inputs=|-+  SaturateOnIntegerOverflow=on
  Out : Outport
  wires:
  _/1 -> Sum/1
  +/1 -> Sum/2
  Sum/1 -> Saturation/1
  Saturation/1 -> Out/1

== system Noordergraaf_Rideout/Systemic/SubSystem1 ==
  + : Inport
  _ : Inport  Port=2
  Saturation : Saturate  UpperLimit=10000  LowerLimit=0
  Sum : Sum  Inputs=|+-  SaturateOnIntegerOverflow=on
  Out : Outport
  wires:
  Saturation/1 -> Out/1
  Sum/1 -> Saturation/1
  _/1 -> Sum/2
  +/1 -> Sum/1

== system Noordergraaf_Rideout/Systemic/SubSystem2 ==
  _1 : Inport
  _2 : Inport  Port=2
  + : Inport  Port=3
  Saturation : Saturate  UpperLimit=10000  LowerLimit=0
  Sum : Sum  Inputs=|--+  SaturateOnIntegerOverflow=on
  Out : Outport
  wires:
  Saturation/1 -> Out/1
  Sum/1 -> Saturation/1
  _1/1 -> Sum/1
  +/1 -> Sum/3
  _2/1 -> Sum/2

== system Noordergraaf_Rideout/Systemic/SubSystem3 ==
  + : Inport
  _ : Inport  Port=2
  Saturation : Saturate  UpperLimit=10000  LowerLimit=0
  Sum : Sum  Inputs=|+-  SaturateOnIntegerOverflow=on
  Out : Outport
  wires:
  +/1 -> Sum/1
  _/1 -> Sum/2
  Sum/1 -> Saturation/1
  Saturation/1 -> Out/1

== system Noordergraaf_Rideout/Control/Left Ventricle/SubSystem1 ==
  _ : Inport
  + : Inport  Port=2
  Saturation : Saturate  UpperLimit=10000  LowerLimit=0
  Sum : Sum  Inputs=|-+  SaturateOnIntegerOverflow=on
  Out : Outport
  wires:
  _/1 -> Sum/1
  +/1 -> Sum/2
  Sum/1 -> Saturation/1
  Saturation/1 -> Out/1

== system Noordergraaf_Rideout/Control/Right Ventricle/SubSystem1 ==
  _ : Inport
  + : Inport  Port=2
  Saturation : Saturate  UpperLimit=10000  LowerLimit=0
  Sum : Sum  Inputs=|-+  SaturateOnIntegerOverflow=on
  Out : Outport
  wires:
  Saturation/1 -> Out/1
  Sum/1 -> Saturation/1
  +/1 -> Sum/2
  _/1 -> Sum/1

== system Noordergraaf_Rideout/Control/phi/SubSystem ==
  In1 : Inport
  Trigger : TriggerPort  VariantControl=(inherit)
  Data Store Write : DataStoreWrite  IndexOptions=Index vector (dialog)  Indices=1  OutputSizes=1
  Scope : Scope
  wires:
  In1/1 -> Data Store Write/1, Scope/1
